simulink model "motor_model_2019"  (R2019b)
settings: Solver=FixedStepAuto  StartTime=0.0  StopTime=70  FixedStep=1e-3  RelTol=1e-3
values from neighbouring files (symbols this model uses):
  bm = estParam(3)    [getParamMotor.m]    (also in getParamMotorFriction.m; getParamMotorKmRm.m = (Km-A*(Km.^2))/(A*Rm))
  Jm = estParam(2)    [getParamMotor.m]    (also in getParamMotorFriction.m; getParamMotorKmRm.m = 4.6e-06)
  Km = double(vpa(sol))    [getParamMotor.m]    (also in getParamMotorFriction.m; getParamMotorKmRm.m = estParam(2))
  Rm = estParam(1)    [getParamMotor.m]    (also in getParamMotorFriction.m; getParamMotorKmRm.m)
undefined symbols (not defined in the file or in its folder): amplM, omegaM
settings Model: Creator=Guido  LastModifiedBy=pietr

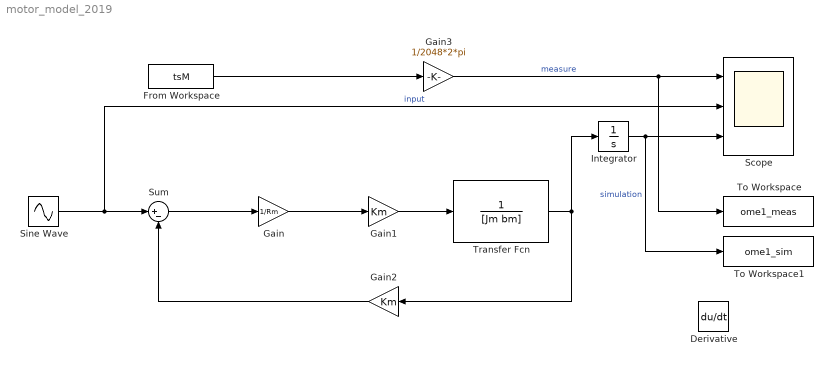
== system motor_model_2019 ==
  Derivative : Derivative
  From Workspace : FromWorkspace  VariableName=tsM  SampleTime=0
  Gain : Gain  Gain=1/Rm
  Gain1 : Gain  Gain=Km
  Gain2 : Gain  Gain=Km
  Gain3 : Gain  Gain=1/2048*2*pi
  Integrator : Integrator
  Scope : Scope  NumInputPorts=3
  Sine Wave : Sin  Amplitude=amplM  Frequency=omegaM  SampleTime=0
  Sum : Sum  Inputs=|+-
  To Workspace : ToWorkspace  VariableName=ome1_meas  SaveFormat=Timeseries  SampleTime=-1
  To Workspace1 : ToWorkspace  VariableName=ome1_sim  SaveFormat=Timeseries  SampleTime=-1
  Transfer Fcn : TransferFcn  Denominator=[Jm bm]
  wires:
  Gain/1 -> Gain1/1
  Gain1/1 -> Transfer Fcn/1
  Sum/1 -> Gain/1
  Gain2/1 -> Sum/2
  Sine Wave/1 -> Scope/2, Sum/1  "input"
  Gain3/1 -> To Workspace/1, Scope/1  "measure"
  From Workspace/1 -> Gain3/1
  Transfer Fcn/1 -> Integrator/1, Gain2/1
  Integrator/1 -> To Workspace1/1, Scope/3  "simulation"
